simulink model "modelforreview3"  (R2021a)
settings: Solver=FixedStepDiscrete  StartTime=0.0  StopTime=5.09  FixedStep=10e-6  RelTol=1e-3
undefined symbols (not defined in the file): DiscIntNeverNeededParam
libraries: spsRMSLib x2, spsCurrentMeasurementLib x1, spsFirstOrderFilterLib x1, spsGroundLib x1, spsPermanentMagnetSynchronousMachineLib x1, spsThreePhaseSeriesRLCBranchLib x1, spsThreePhaseVIMeasurementLib x1, spsVoltageMeasurementLib x1, spsWindTurbineLib x1, spspowerguiLib x1
settings Model: Creator=Aviral  LastModifiedBy=ahele
settings SolverCC: AlgebraicLoopSolver=TrustRegion
settings DebuggingCC: SFMachineParentedDataDiag=warning

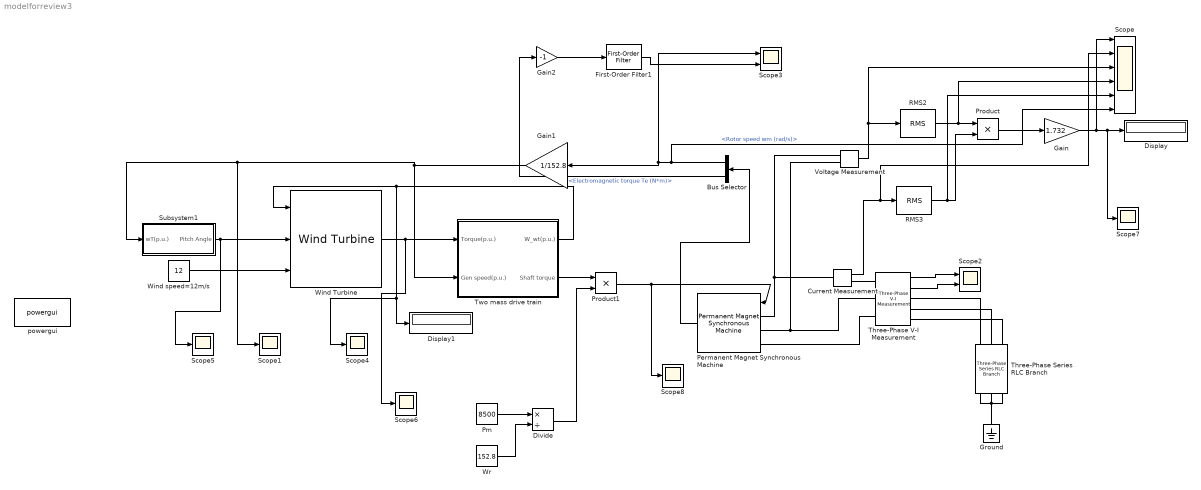
== system modelforreview3 ==
  Bus Selector : BusSelector  OutputSignals=Rotor speed wm (rad/s),Electromagnetic torque Te (N*m)
  Current Measurement : spsCurrentMeasurementLib/Current Measurement  PhasorSimulation=off  OutputType=Complex  PSBequivalent=0
  Display : Display
  Display1 : Display
  Divide : Product  Inputs=*/
  First-Order Filter1 : spsFirstOrderFilterLib/First-Order Filter  FilterType=Lowpass  Tc=1e-3  Ts=50e-6  Initialize=on  Vac_Init=[0, 0, 50]  Vdc_Init=0  PlotResponse=off  FreqRange="[0,  200,  1]"
  Gain : Gain  Gain=1.732
  Gain1 : Gain  Gain=1/152.8
  Gain2 : Gain  Gain=-1
  Ground : spsGroundLib/Ground  LConnTagsString=a
  Permanent Magnet Synchronous Machine : spsPermanentMagnetSynchronousMachineLib/Permanent Magnet Synchronous Machine  NbPhases=3  FluxDistribution=Sinusoidal  RotorType=Round  MechanicalLoad=Torque Tm  PresetModel=No  ShowDetailedParameters=on  MeasurementBus=off  Resistance=0.425  Inductance=8.5e-3  dqInductances=[8.5e-3,8.5e-3]  La=0.000395  MachineConstant=Flux linkage established by magnets (V.s)  Flux=0.433  VoltageCst=392.6876  TorqueCst=3.2475  Flat=120  Mechanical=[0.01197 0.001189 5 0]  PolePairs=4  InitialConditions=[0,0, 0,0]  InitialConditions5ph=[0 0 0 0 0 0]  RefAngle=Aligned with phase A axis (original Park)  IterativeDiscreteModel=Trapezoidal non iterative  TsBlock=-1  TsPowergui=0
  Pm : Constant  Value=8500
  Product : Product
  Product1 : Product
  RMS2 : spsRMSLib/RMS  TrueRMS=on  Freq=50  RMSInit=120  Ts=50e-6
  RMS3 : spsRMSLib/RMS  TrueRMS=on  Freq=50  RMSInit=120  Ts=50e-6
  Scope : Scope  NumInputPorts=6
  Scope{1,4..8} (6 alike) : Scope
  Scope2 : Scope  NumInputPorts=2
  Scope3 : Scope  NumInputPorts=2
  Subsystem1 : Subsystem
  Three-Phase Series RLC Branch : spsThreePhaseSeriesRLCBranchLib/Three-Phase Series RLC Branch  LConnTagsString=A|B|C  RConnTagsString=A|B|C  BranchType=R  Resistance=20  Inductance=1e-3  Capacitance=1e-6  Measurements=None
  Three-Phase V-I Measurement : spsThreePhaseVIMeasurementLib/Three-Phase V-I Measurement  VoltageMeasurement=phase-to-phase  SetLabelV=off  LabelV=Vabc  Vpu=off  VpuLL=off  CurrentMeasurement=yes  SetLabelI=off  LabelI=Iabc  Ipu=off  Pbase=100e6  Vbase=500e3  OutputType=Complex  PhasorSimulation=off  PSBequivalent=0
  Two mass drive train : Subsystem
  Voltage Measurement : spsVoltageMeasurementLib/Voltage Measurement  PhasorSimulation=off  OutputType=Complex  PSBequivalent=0
  Wind Turbine : spsWindTurbineLib/Wind Turbine  Pnom=8.5e3  Pelec_base=8.5e3/0.9  wind_base=12  P_wind_base=0.8  speed_nom=1  pitch_angle=0  c1_c6="[0.51763          116          0.4            5           21     0.006795]"  cp_nom=0.48  lambda_nom=8.1
      settings: SourceProductBaseCode=PS
  Wind speed=12m/s : Constant  Value=12
  Wr : Constant  Value=152.8
  powergui : spspowerguiLib/powergui  Priority=1  SimulationMode=Discrete  SampleTime=20e-6  frequency=60  Iterations=50  frequencyindice=0  Pbase=100e6  ErrMax=1e-4  UnitsV=kV  UnitsW=MW  buscounter=0  FunctionMessages=off  echomessages=off  EnableUseOfTLC=off  CurrentSourceSwitches=off  DisableSnubberDevices=off  DisableRonSwitches=off  DisableVfSwitches=off  DisplayEquations=off  AutomaticDiscreteSolvers=off  SolverType=Tustin/Backward Euler (TBE)  Interpol=off  ExternalGateDelay=off  methode=off  Ts=100  x0status=blocks  SPID=on  SwTol=0  HookPort=off  NonlinearTolerance=1e-4  nMaxIteration=100  ContinueOnMaxIteration=off  RestoreLinks=warning  ResistiveCurrentMeasurement=off  Frange=[0:2:500]  Ylog=off  Xlog=on  ShowGrid=off  save=off  variable=ZData  structure=0  ZoomFFT=off  StartTime=0.0  cycles=1  DisplayStyle=1  fundamental=60  FreqAxis=off  MaxFrequency=1000  frequencyindicesteady=1  RmsSteady=1  display=off
  wires:
  Pm/1 -> Divide/1
  Wr/1 -> Divide/2
  Product1/1 -> Scope8/1, Permanent Magnet Synchronous Machine/1
  Divide/1 -> Product1/2
  Wind Turbine/1 -> Scope6/1, Two mass drive train/1(Torque(p.u.))
  Current Measurement/1 -> Scope/2, RMS3/1
  RMS3/1 -> Scope/5, Product/2
  Product/1 -> Gain/1
  Gain/1 -> Scope7/1, Display/1, Scope/1
  Subsystem1/1(Pitch Angle) -> Scope5/1, Wind Turbine/2
  Wind speed=12m/s/1 -> Wind Turbine/3
  Permanent Magnet Synchronous Machine/1 -> Bus Selector/1
  Bus Selector/1 -> Scope/6, Scope3/1, Gain1/1  "<Rotor speed wm (rad/s)>"
  Gain1/1 -> Two mass drive train/2(Gen speed(p.u.)), Scope1/1, Subsystem1/1(wT(p.u.))
  Two mass drive train/1(W_wt(p.u.)) -> Scope4/1, Display1/1, Wind Turbine/1
  Two mass drive train/2(Shaft torque) -> Product1/1
  Three-Phase V-I Measurement/1 -> Scope2/1
  Three-Phase V-I Measurement/2 -> Scope2/2
  Voltage Measurement/1 -> Scope/3, RMS2/1
  RMS2/1 -> Scope/4, Product/1
  First-Order Filter1/1 -> Scope3/2
  Gain2/1 -> First-Order Filter1/1
  Bus Selector/2 -> Gain2/1  "<Electromagnetic torque Te (N*m)>"
  connections:
  Three-Phase V-I Measurement/LConn1 -- Current Measurement/RConn1
  Permanent Magnet Synchronous Machine/LConn1 -- Voltage Measurement/LConn1 -- Current Measurement/LConn1
  Permanent Magnet Synchronous Machine/LConn2 -- Voltage Measurement/LConn2 -- Three-Phase V-I Measurement/LConn2
  Permanent Magnet Synchronous Machine/LConn3 -- Three-Phase V-I Measurement/LConn3
  Three-Phase V-I Measurement/RConn1 -- Three-Phase Series RLC Branch/LConn1
  Three-Phase V-I Measurement/RConn2 -- Three-Phase Series RLC Branch/LConn2
  Three-Phase V-I Measurement/RConn3 -- Three-Phase Series RLC Branch/LConn3
  Three-Phase Series RLC Branch/RConn1 -- Three-Phase Series RLC Branch/RConn2 -- Ground/LConn1 -- Three-Phase Series RLC Branch/RConn3

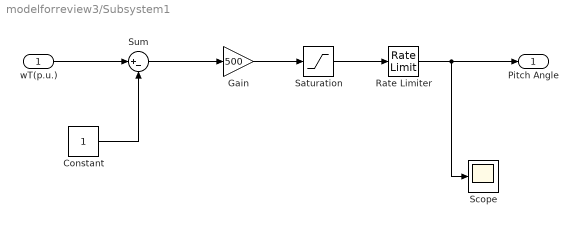
== system modelforreview3/Subsystem1 ==
  wT(p.u.) : Inport
  Constant : Constant
  Gain : Gain  Gain=500
  Rate Limiter : RateLimiter  RisingSlewLimit=2  FallingSlewLimit=-2  SampleTimeMode=inherited
  Saturation : Saturate  UpperLimit=45  LowerLimit=0
  Scope : Scope
  Sum : Sum  Inputs=|+-
  Pitch Angle : Outport
  wires:
  wT(p.u.)/1 -> Sum/1
  Constant/1 -> Sum/2
  Sum/1 -> Gain/1
  Saturation/1 -> Rate Limiter/1
  Gain/1 -> Saturation/1
  Rate Limiter/1 -> Scope/1, Pitch Angle/1

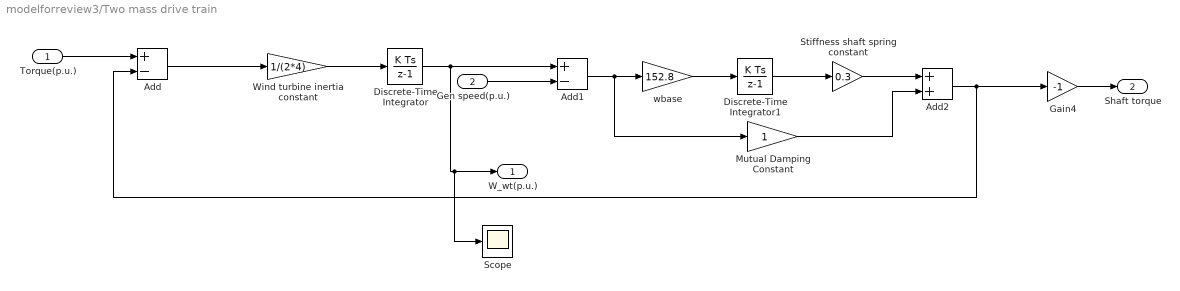
== system modelforreview3/Two mass drive train ==
  Torque(p.u.) : Inport
  Gen speed(p.u.) : Inport  Port=2
  Add : Sum  Inputs=+-
  Add1 : Sum  Inputs=+-
  Add2 : Sum
  Discrete-Time Integrator : DiscreteIntegrator  InitialCondition=1  SampleTime=50e-6  ICPrevOutput=DiscIntNeverNeededParam  ICPrevScaledInput=DiscIntNeverNeededParam
  Discrete-Time Integrator1 : DiscreteIntegrator  InitialCondition=1/0.3  SampleTime=50e-6  ICPrevOutput=DiscIntNeverNeededParam  ICPrevScaledInput=DiscIntNeverNeededParam
  Gain4 : Gain  Gain=-1
  Mutual Damping Constant : Gain
  Scope : Scope
  Stiffness shaft spring constant : Gain  Gain=0.3
  Wind turbine inertia constant : Gain  Gain=1/(2*4)
  wbase : Gain  Gain=152.8
  W_wt(p.u.) : Outport
  Shaft torque : Outport  Port=2
  wires:
  Torque(p.u.)/1 -> Add/1
  Add/1 -> Wind turbine inertia constant/1
  Wind turbine inertia constant/1 -> Discrete-Time Integrator/1
  Discrete-Time Integrator/1 -> Scope/1, W_wt(p.u.)/1, Add1/1
  Gen speed(p.u.)/1 -> Add1/2
  Add1/1 -> Mutual Damping Constant/1, wbase/1
  wbase/1 -> Discrete-Time Integrator1/1
  Discrete-Time Integrator1/1 -> Stiffness shaft spring constant/1
  Stiffness shaft spring constant/1 -> Add2/1
  Mutual Damping Constant/1 -> Add2/2
  Add2/1 -> Gain4/1, Add/2
  Gain4/1 -> Shaft torque/1
